simulink model "usrp_fm_fdm"  (R2014b)
settings: Solver=ode45  StartTime=0.0  StopTime=inf  RelTol=1e-3
PreLoadFcn:
  | %%%%%%%%%%%%%%%%%%%%%%%%%%%%%%%%%%%%%%%%%%%%%%%%%%%%%%%%%%%%%%%%%%%%%%%%%%%
  | % check to see if Simulink library folder is missing from the MATLAB path %
  | %%%%%%%%%%%%%%%%%%%%%%%%%%%%%%%%%%%%%%%%%%%%%%%%%%%%%%%%%%%%%%%%%%%%%%%%%%%
  | if isempty(strfind(path, 'rtlsdr_book_library'))
  | 
  |     % create error window
  |     fig_error = figure(...
  |         'Name', 'Error: RTL-SDR Book Library',...
  |         'Toolbar','none',...
  |         'MenuBar','none',...
  |         'NumberTitle','off',...
  |         'Resize','off',...
  |         'WindowStyle','modal');
  |     fig_error.Position(3) = 600;
  |     fig_error.Position(4) = 150;
  |     fig_axes = axes(...
  |         'Parent',fig_error,...
  |         'Position',[0,0,1,1],...
  |         'visible','off');
  |     % error message
  |     t_title = text(.05,.8,...
  |         'MISSING DIRECTORIES',...
  |         'FontSize',11.5);
  |     t_body = text(.075,.6,...
  |         [{'Simulink cannot find the  \it{<root>}\rm / \it{rtlsdr\_book\_library}\rm  folder in the \it{MATLAB Path}\rm.'},...
  |         {'Please set the MATLAB path following the instructions given in Exercise 2.4.'}],...
  |         'FontSize',10.5);
  |     % buttons
  |     btn_path = uicontrol(...
  |         'Parent',fig_error,...
  |         'String','Set Path Now',...
  |         'FontSize',10,...
  |         'Callback', 'pathtool; close(fig_error);',...
  |         'Position', [fig_error.Position(3)/2-210, 30, 200, 30]);
  |     btn_abort = uicontrol(...
  |         'Parent',fig_error,...
  |         'String','No thanks',...
  |         'FontSize',10,...
  |         'Callback', 'close(fig_error); abort=1;',...
  |         'Position', [fig_error.Position(3)/2+10, 30, 200, 30]);
  | 
  |     % pause to allow user to interact with error box
  |     uiwait(fig_error);
  | 
  |     % abort simulation
  |     try
  |         if abort==1
  |             set_param(gcs, 'SimulationCommand', 'stop');
  |         end
  |     end
  | 
  |     % if user has set path, allow diagram to be updated
  |     if ~exist('abort','var')
  |         % create error window
  |         fig_update = figure(...
  |             'Name', 'Update Diagram',...
  |             'Toolbar','none',...
  |             'MenuBar','none',...
  |             'NumberTitle','off',...
  |             'Resize','off');
  | ... (+24 lines)
undefined symbols (not defined in the file): dfilt, fdesignblkfcn, gcbh, startfcn_spectrum_analyzer
libraries: dsparch4 x9, dspmlti4 x4, dspvision x4, dspsrcs4 x4, dspmtrx3 x2, rtlsdr_book_library x1, commsdrhw_v2 x1
(part 2 of 2)

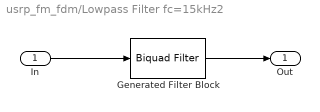
== system usrp_fm_fdm/Lowpass Filter fc=15kHz2 ==
  In : Inport
  Generated Filter Block : dsparch4/Biquad Filter  Tag=BlockMethodSubSystem  IIRFiltStruct=Direct form II  CoeffSource=Specify via dialog  BiQuadCoeffs=[0.47317005345169666 -0.30307728548160168 0.3552862054548247 1 -1.3238737006712475 0.86511185339799446;0.25407991836614779 0.013136135916053305 0.00082836158684250797 1 -1.5734734560410242 0.70525008464109618;0.26098132032063748 -0.29548649035134594 0.034572981551380208 1 -1.3156763282103388 0.66891715813083463;0.030797704742965809 -0.0062470044848620589 0.0024961066929451189 1 -1.3942015618174157 0.77798854949818474;1.5211188179161075 -2 1.5075788908074403 1 -1.3865253012495609 0.98071245573948018;-0.86987276178120643 0.55655777437114651 -0.25149509973734757 1 -1.357338185996994 0.84525618519026846;0.25557566805887638 0.14108303077480563 0.19172424260597029 1 -1.6306553480127399 0.68783931627099504;0.1592819381000054 0.076004983723057917 0.0061187770260567554 1 -1.8253479266443986 0.82545247207677486;0.07934261365834086 -0.0022173795904536437 0.045369159306579282 1 -1.4840124255643086 0.72683648922007227;1.6187100875684302 -2 1.5743866150788544 1 -1.3664078844337517 0.93151058917172236]  a0Flag=Warning  IC=0  ICnum=0  ICden=0  InputProcessing=Columns as channels (frame based)  denAccumFracLength=30  denProdOutputFracLength=30  secondMemoryFracLength=15  roundingMode=Floor  overflowMode=off  ScaleValues=[0.094760439304554744;1;1;1;1;1;1;1;1;1;3.8950302415849745]  optimizeScaleValues=off  ScaleValueMode=Specify via input port (g)  scaleValueFracLength=14  FilterSource=Specify via dialog  dfiltObjectName=dfilt.df2tsos([1 0.3 0.4],[1 0.1 0.2])
  Out : Outport
  wires:
  Generated Filter Block/1 -> Out/1
  In/1 -> Generated Filter Block/1

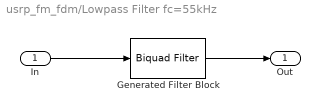
== system usrp_fm_fdm/Lowpass Filter fc=55kHz ==
  In : Inport
  Generated Filter Block : dsparch4/Biquad Filter  Tag=BlockMethodSubSystem  IIRFiltStruct=Direct form II  CoeffSource=Specify via dialog  BiQuadCoeffs=[0.04874889574799169 0.09749779149598338 0.04874889574799169 1 -1.2785946015835052 0.90882045009419532;0.073056637662021584 0.14611327532404317 0.073056637662021584 1 -1.1921933964458502 0.77983164701675012;0.093772917929064087 0.18754583585812817 0.093772917929064087 1 -1.1179521849694893 0.66899656095402338;0.11138436805277892 0.22276873610555784 0.11138436805277892 1 -1.0541562980292758 0.57375535355915264;0.12629559134650412 0.25259118269300823 0.12629559134650412 1 -0.99938424345074539 0.4919858718612854;0.13882982575505176 0.27765965151010352 0.13882982575505176 1 -0.95246064748827952 0.42193339435654365;0.14924961678483584 0.29849923356967167 0.14924961678483584 1 -0.91241591520267207 0.36215040777843066;0.15775884423173145 0.3155176884634629 0.15775884423173145 1 -0.87845250917433237 0.31144626441550949;0.16450679032869461 0.32901358065738923 0.16450679032869461 1 -0.84991723443719058 0.26884580614683345;0.16958371235504627 0.33916742471009254 0.16958371235504627 1 -0.82627875183947086 0.23355579402270807;0.17299233461512931 0.34598466923025861 0.17299233461512931 1 -0.80710954654914568 0.20493798895383786;0.17456113050982916 0.34912226101965832 0.17456113050982916 1 -0.79207165927886913 0.18248784978371677;0.17349234339565367 0.34698468679130734 0.17349234339565367 1 -0.78090559664938042 0.16581797751317565;0.16308101448360895 0.32616202896721791 0.16308101448360895 1 -0.77342195043501816 0.154645603628949;0.10040245645515297 0.20080491291030594 0.10040245645515297 1 -0.76949536305829647 0.14878358115952389;0.095009865630852466 0.19001973126170493 0.095009865630852466 1 -0.76884329378874661 0.14781010359669594;0.095711426494153512 0.19142285298830702 0.095711426494153512 1 -0.77101947868278531 0.15105894120619517;0.096858083734933723 0.19371616746986745 0.096858083734933723 1 -0.77671275156023867 0.15955845753685266;0.098469154776938808 0.19693830955387762 0.098469154776938808 1 -0.78601804909059492 0.17345038403032992;0.10057218773662691 0.20114437547325381 0.10057218773662691 1 -0.79909213509924082 0.19296875420699594;0.10320384479385145 0.20640768958770289 0.10320384479385145 1 -0.81615856673205145 0.21844731767855907;0.10641109543319786 0.21282219086639573 0.10641109543319786 1 -0.83751486314253987 0.25033024231794571;0.1102527707465059 0.2205055414930118 0.1102527707465059 1 -0.86354218882639833 0.28918657055918984;0.11480154369035356 0.22960308738070712 0.11480154369035356 1 -0.89471796702235795 0.33572905000838166;0.12014641411620385 0.24029282823240769 0.12014641411620385 1 -0.93163194980219299 0.39083812456360723;0.12639578958904873 0.25279157917809747 0.12639578958904873 1 -0.97500638446751109 0.45559204093232647;0.13368125928811037 0.26736251857622073 0.13368125928811037 1 -1.025721014860602 0.53130417321679702;0.14216215029377582 0.28432430058755165 0.14216215029377582 1 -1.0848437071413672 0.6195687442938087;0.15203091742706315 0.3040618348541263 0.15203091742706315 1 -1.1536674247472813 0.72231602592238464;0.058820291824625975 0.11764058364925195 0.058820291824625975 1 -1.2337539677586444 0.84187763746689703;0.027752137064996154 0.055504274129992308 0.027752137064996154 1 -1.3269840998317588 0.98106138065316217;0.055172902446354616 0.11034580489270923 0.055172902446354616 1 -1.2557480443196827 0.87471270736993989;0.078740132807287769 0.15748026561457554 0.078740132807287769 1 -1.1725655633060836 0.7505291540750294;0.098969477047013435 0.19793895409402687 0.098969477047013435 1 -1.1010841166201444 0.64381413504753215;0.11632906896976081 0.23265813793952161 0.11632906896976081 1 -1.0396670849263012 0.55212433287247209;0.13116696168000211 0.26233392336000422 0.13116696168000211 1 -0.98695866111014441 0.47343565614264088;0.14379594507760707 0.28759189015521414 0.14379594507760707 1 -0.94183843210645535 0.40607543443631611;0.1544882048274821 0.3089764096549642 0.1544882048274821 1 -0.90338273152428594 0.34866472145267441;0.16339424990042881 0.32678849980085761 0.16339424990042881 1 -0.8708324879516004 ...(+2287 chars)Flag=Warning  IC=0  ICnum=0  ICden=0  InputProcessing=Columns as channels (frame based)  denAccumFracLength=30  denProdOutputFracLength=30  secondMemoryFracLength=15  roundingMode=Floor  overflowMode=off  ScaleValues=[0.067638928049733496;1;1;1;1;1;1;1;1;1;1;1;1;1;1;1;1;1;1;1;1;1;1;1;1;1;1;1;1;1;1;1;1;1;1;1;1;1;1;1;1;1;1;1;1;1;1;1;1;1;1;1;1;1;1;1;1;1;1;1;1;1]  optimizeScaleValues=off  ScaleValueMode=Specify via input port (g)  scaleValueFracLength=14  FilterSource=Specify via dialog  dfiltObjectName=dfilt.df2tsos([1 0.3 0.4],[1 0.1 0.2])
  Out : Outport
  wires:
  Generated Filter Block/1 -> Out/1
  In/1 -> Generated Filter Block/1

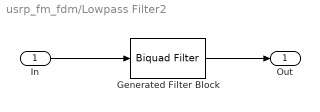
== system usrp_fm_fdm/Lowpass Filter2 ==
  In : Inport
  Generated Filter Block : dsparch4/Biquad Filter  Tag=BlockMethodSubSystem  IIRFiltStruct=Direct form II  CoeffSource=Specify via dialog  BiQuadCoeffs=[0.02505658453151734 0.050113169063034681 0.02505658453151734 1 -1.6618358052504689 0.92327518660477159;0.037716014607021689 0.075432029214043378 0.037716014607021689 1 -1.5666197180702381 0.81307974054400167;0.048494542600695072 0.096989085201390143 0.048494542600695072 1 -1.483833787366122 0.71726995848240305;0.057562689362794101 0.1151253787255882 0.057562689362794101 1 -1.4124095756411101 0.63460931673938947;0.065066669960849324 0.13013333992169865 0.065066669960849324 1 -1.3513355886493104 0.5639271931762575;0.071126049882347511 0.14225209976469502 0.071126049882347511 1 -1.2996951874675289 0.50416274358054824;0.075826965263644491 0.15165393052728898 0.075826965263644491 1 -1.2566848480829704 0.45438603384519421;0.079207708097762716 0.15841541619552543 0.079207708097762716 1 -1.2216205877683222 0.41380547733850032;0.081213644661423695 0.16242728932284739 0.081213644661423695 1 -1.1939377721788489 0.38176761165383055;0.08148106483340975 0.1629621296668195 0.08148106483340975 1 -1.1731876770814522 0.35775311943117882;0.076637308661870573 0.15327461732374115 0.076637308661870573 1 -1.1590329311748637 0.34137155424355531;0.047546496662289287 0.095092993324578573 0.047546496662289287 1 -1.1512431451247189 0.3323562819935113;0.04540058431321875 0.090801168626437501 0.04540058431321875 1 -1.1496915016555413 0.3305605345596806;0.045831247000341468 0.091662494000682937 0.045831247000341468 1 -1.1543527405881076 0.3359550778409825;0.046516257123944797 0.093032514247889594 0.046516257123944797 1 -1.1653027462029997 0.34862773420436555;0.047466760014933662 0.094933520029867324 0.047466760014933662 1 -1.1827197756415799 0.36878480413735909;0.048698191344618065 0.09739638268923613 0.048698191344618065 1 -1.2068872094697505 0.39675424952948513;0.050230457593599342 0.10046091518719868 0.050230457593599342 1 -1.2381975142107695 0.43299027958924174;0.052088101393404251 0.1041762027868085 0.052088101393404251 1 -1.2771568309371673 0.47807866131156473;0.054300385989436643 0.10860077197887329 0.054300385989436643 1 -1.3243891792379572 0.53274158481157419;0.056901193140924844 0.11380238628184969 0.056901193140924844 1 -1.3806386047689676 0.59784014872671409;0.059928568932260555 0.11985713786452111 0.059928568932260555 1 -1.4467665832625731 0.6743713558262725;0.063423665332839996 0.12684733066567999 0.063423665332839996 1 -1.5237404723519465 0.76345474808098879;0.023993836801624483 0.047987673603248966 0.023993836801624483 1 -1.612606599730263 0.86630126106162297;0.014199710532717848 0.028399421065435696 0.014199710532717848 1 -1.7144385404499303 0.98415336424243371;0.028453803345255303 0.056907606690510606 0.028453803345255303 1 -1.6368075882726612 0.89430953998294882;0.04083171761385794 0.08166343522771588 0.04083171761385794 1 -1.5448001049050344 0.78782747407497666;0.051459392354549008 0.10291878470909802 0.051459392354549008 1 -1.4649534370622368 0.69541935859814075;0.060531990296125222 0.12106398059225044 0.060531990296125222 1 -1.3962083671487442 0.61585934024476119;0.06815377125244737 0.13630754250489474 0.06815377125244737 1 -1.3375744913620335 0.54800120526008977;0.074455848419753085 0.14891169683950617 0.074455848419753085 1 -1.2881623105057174 0.49081551877004753;0.079552479596548167 0.15910495919309633 0.079552479596548167 1 -1.2471979145071224 0.44340661946156557;0.083510197687583193 0.16702039537516639 0.083510197687583193 1 -1.2140273488611264 0.40501767295371627;0.086395360489223874 0.17279072097844775 0.086395360489223874 1 -1.1881153515668013 0.37502921002970635;0.08825814050628647 0.17651628101257294 0.08825814050628647 1 -1.1690414739763555 0.35295463721924042;0.072653340568011524 0.14530668113602305 0.072653340568011524 1 -1.1564954726095342 0.33843490365490059;0.10631278825624907 0.21262557651249814 0.10631278825624907 1 -1.150273121708774 0.33123365486006179;0.09066349956390464 0.09066349956390464 0 1 -0.57474884697500372 0;0.045700079748393248 0.091400159496786496 0.045700079748393248 1 -1.1526025576110279 ...(+1167 chars)Flag=Warning  IC=0  ICnum=0  ICden=0  InputProcessing=Columns as channels (frame based)  denAccumFracLength=30  denProdOutputFracLength=30  secondMemoryFracLength=15  roundingMode=Floor  overflowMode=off  ScaleValues=[0.038531123333914737;1;1;1;1;1;1;1;1;1;1;1;1;1;1;1;1;1;1;1;1;1;1;1;1;1;1;1;1;1;1;1;1;1;1;1;1;1;1;1;1;1;1;1;1;1;1;1;1;1;1]  optimizeScaleValues=off  ScaleValueMode=Specify via input port (g)  scaleValueFracLength=14  FilterSource=Specify via dialog  dfiltObjectName=dfilt.df2tsos([1 0.3 0.4],[1 0.1 0.2])
  Out : Outport
  wires:
  Generated Filter Block/1 -> Out/1
  In/1 -> Generated Filter Block/1

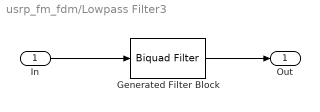
== system usrp_fm_fdm/Lowpass Filter3 ==
  In : Inport
  Generated Filter Block : dsparch4/Biquad Filter  Tag=BlockMethodSubSystem  IIRFiltStruct=Direct form II  CoeffSource=Specify via dialog  BiQuadCoeffs=[0.02505658453151734 0.050113169063034681 0.02505658453151734 1 -1.6618358052504689 0.92327518660477159;0.037716014607021689 0.075432029214043378 0.037716014607021689 1 -1.5666197180702381 0.81307974054400167;0.048494542600695072 0.096989085201390143 0.048494542600695072 1 -1.483833787366122 0.71726995848240305;0.057562689362794101 0.1151253787255882 0.057562689362794101 1 -1.4124095756411101 0.63460931673938947;0.065066669960849324 0.13013333992169865 0.065066669960849324 1 -1.3513355886493104 0.5639271931762575;0.071126049882347511 0.14225209976469502 0.071126049882347511 1 -1.2996951874675289 0.50416274358054824;0.075826965263644491 0.15165393052728898 0.075826965263644491 1 -1.2566848480829704 0.45438603384519421;0.079207708097762716 0.15841541619552543 0.079207708097762716 1 -1.2216205877683222 0.41380547733850032;0.081213644661423695 0.16242728932284739 0.081213644661423695 1 -1.1939377721788489 0.38176761165383055;0.08148106483340975 0.1629621296668195 0.08148106483340975 1 -1.1731876770814522 0.35775311943117882;0.076637308661870573 0.15327461732374115 0.076637308661870573 1 -1.1590329311748637 0.34137155424355531;0.047546496662289287 0.095092993324578573 0.047546496662289287 1 -1.1512431451247189 0.3323562819935113;0.04540058431321875 0.090801168626437501 0.04540058431321875 1 -1.1496915016555413 0.3305605345596806;0.045831247000341468 0.091662494000682937 0.045831247000341468 1 -1.1543527405881076 0.3359550778409825;0.046516257123944797 0.093032514247889594 0.046516257123944797 1 -1.1653027462029997 0.34862773420436555;0.047466760014933662 0.094933520029867324 0.047466760014933662 1 -1.1827197756415799 0.36878480413735909;0.048698191344618065 0.09739638268923613 0.048698191344618065 1 -1.2068872094697505 0.39675424952948513;0.050230457593599342 0.10046091518719868 0.050230457593599342 1 -1.2381975142107695 0.43299027958924174;0.052088101393404251 0.1041762027868085 0.052088101393404251 1 -1.2771568309371673 0.47807866131156473;0.054300385989436643 0.10860077197887329 0.054300385989436643 1 -1.3243891792379572 0.53274158481157419;0.056901193140924844 0.11380238628184969 0.056901193140924844 1 -1.3806386047689676 0.59784014872671409;0.059928568932260555 0.11985713786452111 0.059928568932260555 1 -1.4467665832625731 0.6743713558262725;0.063423665332839996 0.12684733066567999 0.063423665332839996 1 -1.5237404723519465 0.76345474808098879;0.023993836801624483 0.047987673603248966 0.023993836801624483 1 -1.612606599730263 0.86630126106162297;0.014199710532717848 0.028399421065435696 0.014199710532717848 1 -1.7144385404499303 0.98415336424243371;0.028453803345255303 0.056907606690510606 0.028453803345255303 1 -1.6368075882726612 0.89430953998294882;0.04083171761385794 0.08166343522771588 0.04083171761385794 1 -1.5448001049050344 0.78782747407497666;0.051459392354549008 0.10291878470909802 0.051459392354549008 1 -1.4649534370622368 0.69541935859814075;0.060531990296125222 0.12106398059225044 0.060531990296125222 1 -1.3962083671487442 0.61585934024476119;0.06815377125244737 0.13630754250489474 0.06815377125244737 1 -1.3375744913620335 0.54800120526008977;0.074455848419753085 0.14891169683950617 0.074455848419753085 1 -1.2881623105057174 0.49081551877004753;0.079552479596548167 0.15910495919309633 0.079552479596548167 1 -1.2471979145071224 0.44340661946156557;0.083510197687583193 0.16702039537516639 0.083510197687583193 1 -1.2140273488611264 0.40501767295371627;0.086395360489223874 0.17279072097844775 0.086395360489223874 1 -1.1881153515668013 0.37502921002970635;0.08825814050628647 0.17651628101257294 0.08825814050628647 1 -1.1690414739763555 0.35295463721924042;0.072653340568011524 0.14530668113602305 0.072653340568011524 1 -1.1564954726095342 0.33843490365490059;0.10631278825624907 0.21262557651249814 0.10631278825624907 1 -1.150273121708774 0.33123365486006179;0.09066349956390464 0.09066349956390464 0 1 -0.57474884697500372 0;0.045700079748393248 0.091400159496786496 0.045700079748393248 1 -1.1526025576110279 ...(+1167 chars)Flag=Warning  IC=0  ICnum=0  ICden=0  InputProcessing=Columns as channels (frame based)  denAccumFracLength=30  denProdOutputFracLength=30  secondMemoryFracLength=15  roundingMode=Floor  overflowMode=off  ScaleValues=[0.038531123333914737;1;1;1;1;1;1;1;1;1;1;1;1;1;1;1;1;1;1;1;1;1;1;1;1;1;1;1;1;1;1;1;1;1;1;1;1;1;1;1;1;1;1;1;1;1;1;1;1;1;1]  optimizeScaleValues=off  ScaleValueMode=Specify via input port (g)  scaleValueFracLength=14  FilterSource=Specify via dialog  dfiltObjectName=dfilt.df2tsos([1 0.3 0.4],[1 0.1 0.2])
  Out : Outport
  wires:
  In/1 -> Generated Filter Block/1
  Generated Filter Block/1 -> Out/1

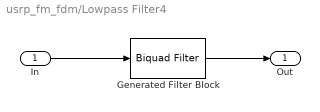
== system usrp_fm_fdm/Lowpass Filter4 ==
  In : Inport
  Generated Filter Block : dsparch4/Biquad Filter  Tag=BlockMethodSubSystem  IIRFiltStruct=Direct form II  CoeffSource=Specify via dialog  BiQuadCoeffs=[0.02505658453151734 0.050113169063034681 0.02505658453151734 1 -1.6618358052504689 0.92327518660477159;0.037716014607021689 0.075432029214043378 0.037716014607021689 1 -1.5666197180702381 0.81307974054400167;0.048494542600695072 0.096989085201390143 0.048494542600695072 1 -1.483833787366122 0.71726995848240305;0.057562689362794101 0.1151253787255882 0.057562689362794101 1 -1.4124095756411101 0.63460931673938947;0.065066669960849324 0.13013333992169865 0.065066669960849324 1 -1.3513355886493104 0.5639271931762575;0.071126049882347511 0.14225209976469502 0.071126049882347511 1 -1.2996951874675289 0.50416274358054824;0.075826965263644491 0.15165393052728898 0.075826965263644491 1 -1.2566848480829704 0.45438603384519421;0.079207708097762716 0.15841541619552543 0.079207708097762716 1 -1.2216205877683222 0.41380547733850032;0.081213644661423695 0.16242728932284739 0.081213644661423695 1 -1.1939377721788489 0.38176761165383055;0.08148106483340975 0.1629621296668195 0.08148106483340975 1 -1.1731876770814522 0.35775311943117882;0.076637308661870573 0.15327461732374115 0.076637308661870573 1 -1.1590329311748637 0.34137155424355531;0.047546496662289287 0.095092993324578573 0.047546496662289287 1 -1.1512431451247189 0.3323562819935113;0.04540058431321875 0.090801168626437501 0.04540058431321875 1 -1.1496915016555413 0.3305605345596806;0.045831247000341468 0.091662494000682937 0.045831247000341468 1 -1.1543527405881076 0.3359550778409825;0.046516257123944797 0.093032514247889594 0.046516257123944797 1 -1.1653027462029997 0.34862773420436555;0.047466760014933662 0.094933520029867324 0.047466760014933662 1 -1.1827197756415799 0.36878480413735909;0.048698191344618065 0.09739638268923613 0.048698191344618065 1 -1.2068872094697505 0.39675424952948513;0.050230457593599342 0.10046091518719868 0.050230457593599342 1 -1.2381975142107695 0.43299027958924174;0.052088101393404251 0.1041762027868085 0.052088101393404251 1 -1.2771568309371673 0.47807866131156473;0.054300385989436643 0.10860077197887329 0.054300385989436643 1 -1.3243891792379572 0.53274158481157419;0.056901193140924844 0.11380238628184969 0.056901193140924844 1 -1.3806386047689676 0.59784014872671409;0.059928568932260555 0.11985713786452111 0.059928568932260555 1 -1.4467665832625731 0.6743713558262725;0.063423665332839996 0.12684733066567999 0.063423665332839996 1 -1.5237404723519465 0.76345474808098879;0.023993836801624483 0.047987673603248966 0.023993836801624483 1 -1.612606599730263 0.86630126106162297;0.014199710532717848 0.028399421065435696 0.014199710532717848 1 -1.7144385404499303 0.98415336424243371;0.028453803345255303 0.056907606690510606 0.028453803345255303 1 -1.6368075882726612 0.89430953998294882;0.04083171761385794 0.08166343522771588 0.04083171761385794 1 -1.5448001049050344 0.78782747407497666;0.051459392354549008 0.10291878470909802 0.051459392354549008 1 -1.4649534370622368 0.69541935859814075;0.060531990296125222 0.12106398059225044 0.060531990296125222 1 -1.3962083671487442 0.61585934024476119;0.06815377125244737 0.13630754250489474 0.06815377125244737 1 -1.3375744913620335 0.54800120526008977;0.074455848419753085 0.14891169683950617 0.074455848419753085 1 -1.2881623105057174 0.49081551877004753;0.079552479596548167 0.15910495919309633 0.079552479596548167 1 -1.2471979145071224 0.44340661946156557;0.083510197687583193 0.16702039537516639 0.083510197687583193 1 -1.2140273488611264 0.40501767295371627;0.086395360489223874 0.17279072097844775 0.086395360489223874 1 -1.1881153515668013 0.37502921002970635;0.08825814050628647 0.17651628101257294 0.08825814050628647 1 -1.1690414739763555 0.35295463721924042;0.072653340568011524 0.14530668113602305 0.072653340568011524 1 -1.1564954726095342 0.33843490365490059;0.10631278825624907 0.21262557651249814 0.10631278825624907 1 -1.150273121708774 0.33123365486006179;0.09066349956390464 0.09066349956390464 0 1 -0.57474884697500372 0;0.045700079748393248 0.091400159496786496 0.045700079748393248 1 -1.1526025576110279 ...(+1167 chars)Flag=Warning  IC=0  ICnum=0  ICden=0  InputProcessing=Columns as channels (frame based)  denAccumFracLength=30  denProdOutputFracLength=30  secondMemoryFracLength=15  roundingMode=Floor  overflowMode=off  ScaleValues=[0.038531123333914737;1;1;1;1;1;1;1;1;1;1;1;1;1;1;1;1;1;1;1;1;1;1;1;1;1;1;1;1;1;1;1;1;1;1;1;1;1;1;1;1;1;1;1;1;1;1;1;1;1;1]  optimizeScaleValues=off  ScaleValueMode=Specify via input port (g)  scaleValueFracLength=14  FilterSource=Specify via dialog  dfiltObjectName=dfilt.df2tsos([1 0.3 0.4],[1 0.1 0.2])
  Out : Outport
  wires:
  Generated Filter Block/1 -> Out/1
  In/1 -> Generated Filter Block/1
